simulink model "mountain_uav_model"  (R2025b)
settings: Solver=FixedStepDiscrete  StartTime=0.0  StopTime=25  FixedStep=0.1  RelTol=1e-3
values from neighbouring files (symbols this model uses):
  OBSTACLES_RH = zeros(N, 2)    [build_mountain_uav_model.m]
  OBSTACLES_XYZ = zeros(N, 3)    [build_mountain_uav_model.m]
undefined symbols (not defined in the file or in its folder): CAM_INTRIN, CAMERA_NOISE_LEVEL, FOG_DENSITY_PERCENT, ILLUMINATION_LUX, IMG_SIZE, UAV_V_VEC, UAV_X0_VEC
settings Model: Creator=lab  LastModifiedBy=lab

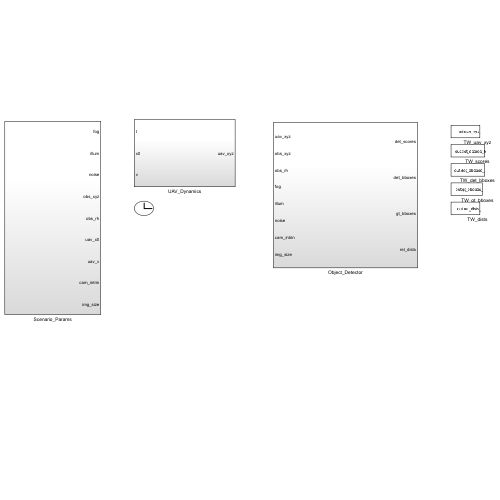
[thumbnail: Simulink's stored preview of the top-level diagram]
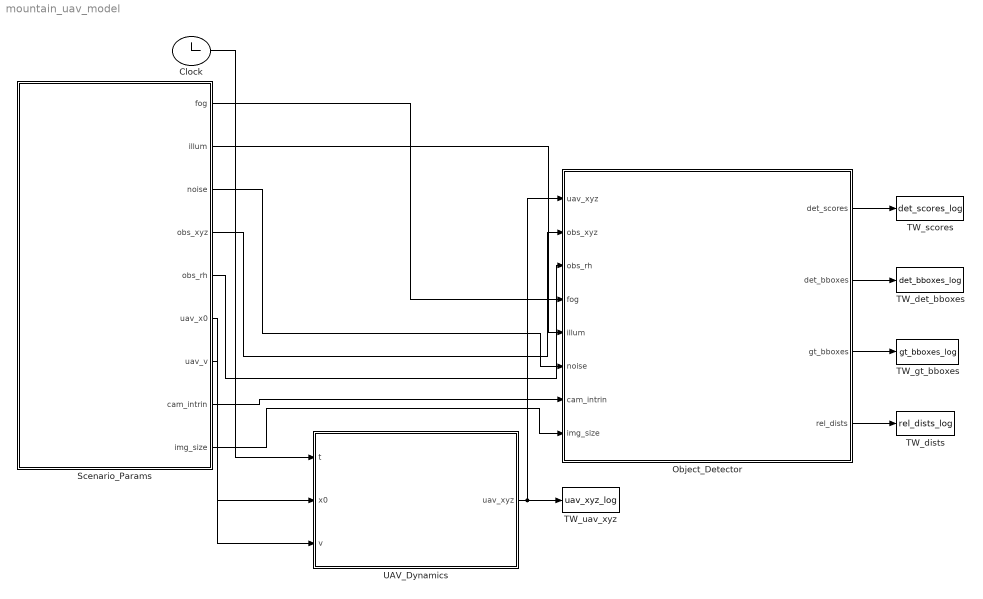
== system mountain_uav_model ==
  Clock : Clock
  Object_Detector : Subsystem
  Scenario_Params : Subsystem
  TW_det_bboxes : ToWorkspace  VariableName=det_bboxes_log  SaveFormat=Structure With Time  SampleTime=-1
  TW_dists : ToWorkspace  VariableName=rel_dists_log  SaveFormat=Structure With Time  SampleTime=-1
  TW_gt_bboxes : ToWorkspace  VariableName=gt_bboxes_log  SaveFormat=Structure With Time  SampleTime=-1
  TW_scores : ToWorkspace  VariableName=det_scores_log  SaveFormat=Structure With Time  SampleTime=-1
  TW_uav_xyz : ToWorkspace  VariableName=uav_xyz_log  SaveFormat=Structure With Time  SampleTime=-1
  UAV_Dynamics : Subsystem
  wires:
  Clock/1 -> UAV_Dynamics/1(t)
  Scenario_Params/2(illum) -> Object_Detector/5(illum)
  Scenario_Params/1(fog) -> Object_Detector/4(fog)
  Object_Detector/3(gt_bboxes) -> TW_gt_bboxes/1
  Scenario_Params/3(noise) -> Object_Detector/6(noise)
  Scenario_Params/5(obs_rh) -> Object_Detector/3(obs_rh)
  Scenario_Params/4(obs_xyz) -> Object_Detector/2(obs_xyz)
  Scenario_Params/7(uav_v) -> UAV_Dynamics/3(v)
  Scenario_Params/6(uav_x0) -> UAV_Dynamics/2(x0)
  Scenario_Params/8(cam_intrin) -> Object_Detector/7(cam_intrin)
  Scenario_Params/9(img_size) -> Object_Detector/8(img_size)
  UAV_Dynamics/1(uav_xyz) -> Object_Detector/1(uav_xyz), TW_uav_xyz/1
  Object_Detector/1(det_scores) -> TW_scores/1
  Object_Detector/2(det_bboxes) -> TW_det_bboxes/1
  Object_Detector/4(rel_dists) -> TW_dists/1

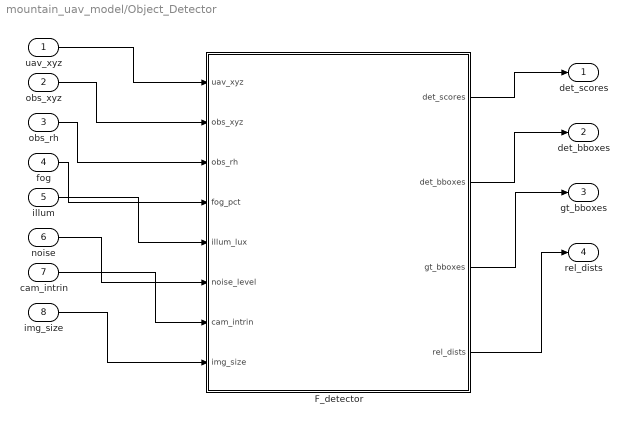
== system mountain_uav_model/Object_Detector ==
  uav_xyz : Inport
  obs_xyz : Inport  Port=2
  obs_rh : Inport  Port=3
  fog : Inport  Port=4
  illum : Inport  Port=5
  noise : Inport  Port=6
  cam_intrin : Inport  Port=7
  img_size : Inport  Port=8
  F_detector : MATLAB Function  TreatAsAtomicUnit=on
  det_scores : Outport
  det_bboxes : Outport  Port=2
  gt_bboxes : Outport  Port=3
  rel_dists : Outport  Port=4
  wires:
  ? -> ?
  uav_xyz/1 -> F_detector/1(uav_xyz)
  obs_xyz/1 -> F_detector/2(obs_xyz)
  obs_rh/1 -> F_detector/3(obs_rh)
  fog/1 -> F_detector/4(fog_pct)
  illum/1 -> F_detector/5(illum_lux)
  noise/1 -> F_detector/6(noise_level)
  cam_intrin/1 -> F_detector/7(cam_intrin)
  img_size/1 -> F_detector/8(img_size)
  F_detector/1(det_scores) -> det_scores/1
  F_detector/2(det_bboxes) -> det_bboxes/1
  F_detector/3(gt_bboxes) -> gt_bboxes/1
  F_detector/4(rel_dists) -> rel_dists/1

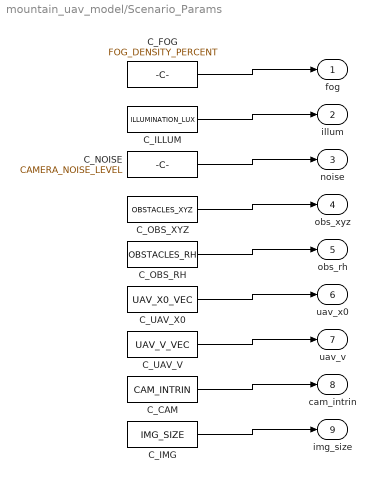
== system mountain_uav_model/Scenario_Params ==
  C_CAM : Constant  Value=CAM_INTRIN  OutDataTypeStr=double
  C_FOG : Constant  Value=FOG_DENSITY_PERCENT  OutDataTypeStr=double
  C_ILLUM : Constant  Value=ILLUMINATION_LUX  OutDataTypeStr=double
  C_IMG : Constant  Value=IMG_SIZE  OutDataTypeStr=double
  C_NOISE : Constant  Value=CAMERA_NOISE_LEVEL  OutDataTypeStr=double
  C_OBS_RH : Constant  Value=OBSTACLES_RH  OutDataTypeStr=double
  C_OBS_XYZ : Constant  Value=OBSTACLES_XYZ  OutDataTypeStr=double
  C_UAV_V : Constant  Value=UAV_V_VEC  OutDataTypeStr=double
  C_UAV_X0 : Constant  Value=UAV_X0_VEC  OutDataTypeStr=double
  fog : Outport
  illum : Outport  Port=2
  noise : Outport  Port=3
  obs_xyz : Outport  Port=4
  obs_rh : Outport  Port=5
  uav_x0 : Outport  Port=6
  uav_v : Outport  Port=7
  cam_intrin : Outport  Port=8
  img_size : Outport  Port=9
  wires:
  ? -> ?
  C_FOG/1 -> fog/1
  C_ILLUM/1 -> illum/1
  C_NOISE/1 -> noise/1
  C_OBS_XYZ/1 -> obs_xyz/1
  C_OBS_RH/1 -> obs_rh/1
  C_UAV_X0/1 -> uav_x0/1
  C_UAV_V/1 -> uav_v/1
  C_CAM/1 -> cam_intrin/1
  C_IMG/1 -> img_size/1

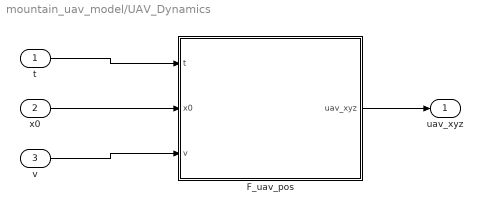
== system mountain_uav_model/UAV_Dynamics ==
  t : Inport
  x0 : Inport  Port=2
  v : Inport  Port=3
  F_uav_pos : MATLAB Function  TreatAsAtomicUnit=on
  uav_xyz : Outport
  wires:
  ? -> ?
  t/1 -> F_uav_pos/1(t)
  x0/1 -> F_uav_pos/2(x0)
  v/1 -> F_uav_pos/3(v)
  F_uav_pos/1(uav_xyz) -> uav_xyz/1

== matlab function mountain_uav_model/Object_Detector/F_detector ==
  data: uav_xyz input; det_scores output; obs_xyz input; obs_rh input; fog_pct input; illum_lux input; noise_level input; cam_intrin input; img_size input; det_bboxes output; gt_bboxes output; rel_dists output
function [det_scores, det_bboxes, gt_bboxes, rel_dists] = F_detector(uav_xyz, obs_xyz, obs_rh, fog_pct, illum_lux, noise_level, cam_intrin, img_size)
%#codegen
% obs_xyz: 5x3, obs_rh: 5x2 (radius, height)
% Returns geometry-projected bboxes (gt) plus weather-degraded detector outputs.

N = size(obs_xyz, 1);
det_scores = zeros(N, 1);
det_bboxes = zeros(N, 4);
gt_bboxes  = zeros(N, 4);
rel_dists  = zeros(N, 1);

fx = cam_intrin(1); fy = cam_intrin(2); cx0 = cam_intrin(3); cy0 = cam_intrin(4);
pitch = cam_intrin(5) * pi/180;
sp = sin(pitch); cp = cos(pitch);
img_w = img_size(1); img_h = img_size(2);

% Weather visibility (shared across obstacles)
fog_norm   = max(0, min(1, fog_pct / 100));
low_light  = max(0, (3000 - illum_lux) / 3000);
high_light = max(0, (illum_lux - 12000) / 12000);
visibility = max(0, 1 - 0.6*fog_norm - 0.20*low_light - 0.10*high_light - 0.20*noise_level);

for k = 1:N
    base_x = obs_xyz(k,1); base_y = obs_xyz(k,2); base_z = obs_xyz(k,3);
    r = obs_rh(k,1); h = obs_rh(k,2);

    dx = base_x - uav_xyz(1);
    dy = base_y - uav_xyz(2);
    dz_base = base_z - uav_xyz(3);
    dz_top  = (base_z + h) - uav_xyz(3);

    rel_dists(k) = sqrt(dx*dx + dy*dy + (dz_base + h/2)^2);

    % Camera looks +X then pitched down by 'pitch' rad (around Y axis).
    % Camera frame in world:
    %   z_c (forward) = ( cos(p), 0, -sin(p) )
    %   x_c (right)   = ( 0,      1,  0      )
    %   y_c (down)    = (-sin(p), 0, -cos(p) )
    % cam_x =  dy ; cam_y = -dx*sp - dz*cp ; cam_z = dx*cp - dz*sp
    cz_base = dx*cp - dz_base*sp;
    cz_top  = dx*cp - dz_top *sp;
    if cz_base < 0.5 || cz_top < 0.5
        continue;
    end
    cz_avg = 0.5*(cz_base + cz_top);

    cam_x_left  = dy - r;
    cam_x_right = dy + r;
    % Box-shaped bbox: include along-x extent (length L = 2r) in vertical
    % projection so the bbox tightly encloses elongated objects (vehicles)
    % at high pitch. Front-top corner = smallest v (highest in image);
    % back-bot corner = largest v (lowest in image).
    cam_y_top   = -dx*sp - r*sp - dz_top *cp;   % front-top corner
    cam_y_bot   = -dx*sp + r*sp - dz_base*cp;   % back-bot corner

    u_left  = fx * cam_x_left  / cz_avg + cx0;
    u_right = fx * cam_x_right / cz_avg + cx0;
    v_top   = fy * cam_y_top   / cz_top  + cy0;
    v_bot   = fy * cam_y_bot   / cz_base + cy0;

    bbox_u = u_left;
    bbox_v = v_top;
    bbox_w = u_right - u_left;
    bbox_h = v_bot - v_top;

    if bbox_w <= 0 || bbox_h <= 0
        continue;
    end

    % Reject if entirely outside image
    if u_right < 0 || u_left > img_w || v_bot < 0 || v_top > img_h
        continue;
    end

    % Reject if too far (extended for higher-altitude surveillance)
    if cz_avg > 150
        continue;
    end

    gt_bboxes(k,:) = [bbox_u, bbox_v, bbox_w, bbox_h];

    dist_attn = max(0.05, 1 - cz_avg/150);
    sc = visibility * dist_attn;

    % Deterministic jitter (no randn in codegen). Scaled to bbox size so
    % it never exceeds ~20% of the bbox in clean conditions; this keeps
    % IoU>=0.5 achievable for small (5-15 px) intruder bboxes.
    seed     = mod(uav_xyz(1)*0.7 + base_x*1.3 + base_y*0.9, 6.2831853);
    bb_size  = 0.5 * (bbox_w + bbox_h);
    pos_amp  = bb_size * 0.10 + bb_size * 0.40 * (1 - visibility);
    size_amp = bb_size * 0.05 + bb_size * 0.25 * (1 - visibility);
    jx = sin(seed)        * pos_amp;
    jy = cos(seed*1.3)    * pos_amp;
    jw = sin(seed*1.7)    * size_amp;
    jh = cos(seed*2.1)    * size_amp;

    det_bboxes(k,:) = [bbox_u + jx, bbox_v + jy, max(2, bbox_w + jw), max(2, bbox_h + jh)];
    det_scores(k)   = sc;
end
end

== matlab function mountain_uav_model/UAV_Dynamics/F_uav_pos ==
  data: t input; uav_xyz output; x0 input; v input
function uav_xyz = F_uav_pos(t, x0, v)
%#codegen
uav_xyz = x0 + t .* v;
end
